simulink model "Temperature_change_in_water_tank"  (R2024b)
settings: Solver=VariableStepAuto  StartTime=0.0  StopTime=10.0  RelTol=1e-3

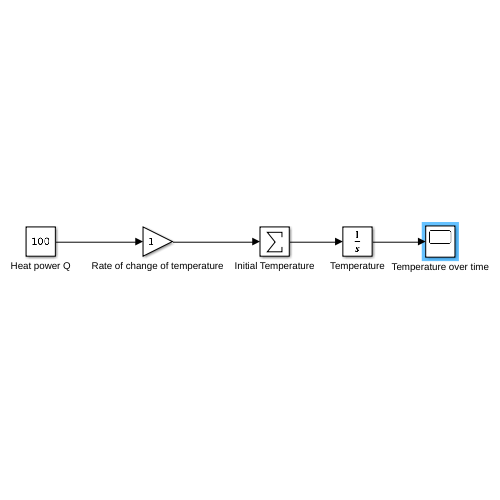
[thumbnail: Simulink's stored preview of the top-level diagram]
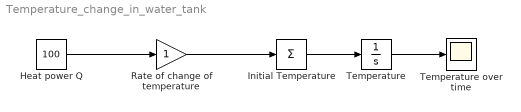
== system Temperature_change_in_water_tank ==
  Heat power Q : Constant  Value=100
  Initial Temperature : Sum  Inputs=+
  Rate of change of temperature : Gain
  Temperature : Integrator
  Temperature over time : Scope
  wires:
  Temperature/1 -> Temperature over time/1
  Heat power Q/1 -> Rate of change of temperature/1
  Rate of change of temperature/1 -> Initial Temperature/1
  Initial Temperature/1 -> Temperature/1
